simulink model "spike_generator_sim"  (R2020b)
settings: Solver=FixedStepDiscrete  StartTime=0.0  StopTime=stopTime  RelTol=1e-3
values from neighbouring files (symbols this model uses):
  nSites = 4    [modelparameters.m]
  tabs = 10e-3    (= 0.01)    [modelparameters.m]
  trel = 10e-3    (= 0.01)    [modelparameters.m]
undefined symbols (not defined in the file or in its folder): mp
libraries: dspsrcs4 x1
settings Model: Creator=Ross  LastModifiedBy=tyler
settings SolverCC: AutoInsertRateTranBlk=on
settings DataIOCC: ReturnWorkspaceOutputs=off
settings OptimizationCC: BlockReduction=off  ConditionallyExecuteInputs=off  DefaultParameterBehavior=Inlined
settings DebuggingCC: ReadBeforeWriteMsg=DisableAll  WriteAfterWriteMsg=DisableAll  WriteAfterReadMsg=DisableAll  AlgebraicLoopMsg=error  MultiTaskDSMMsg=none  SingleTaskRateTransMsg=error  PregeneratedLibrarySubsystemCodeDiagnostic=none  ArithmeticOperatorsInVariantConditions=warning
settings HardwareCC: ProdBitPerPointer=32  ProdBitPerSizeT=32  ProdBitPerPtrDiffT=32  ProdLargestAtomicFloat=None  ProdIntDivRoundTo=Undefined  ProdEndianess=Unspecified  ProdWordSize=32  ProdHWDeviceType=ASIC/FPGA->ASIC/FPGA  TargetBitPerPointer=64  TargetBitPerSizeT=64  TargetBitPerPtrDiffT=64  TargetLongLongMode=on  TargetIntDivRoundTo=Zero  TargetEndianess=LittleEndian  TargetWordSize=64  TargetHWDeviceType=Custom Processor->MATLAB Host Computer  ProdEqTarget=off
settings ModelReferenceCC: UpdateModelReferenceTargets=IfOutOfDate
settings SFSimCC: SFSimEcho=off  SimUseLocalCustomCode=off  CustomCodeUndefinedFunction=UseInterfaceOnly
settings RTWCC: RTWUseLocalCustomCode=off

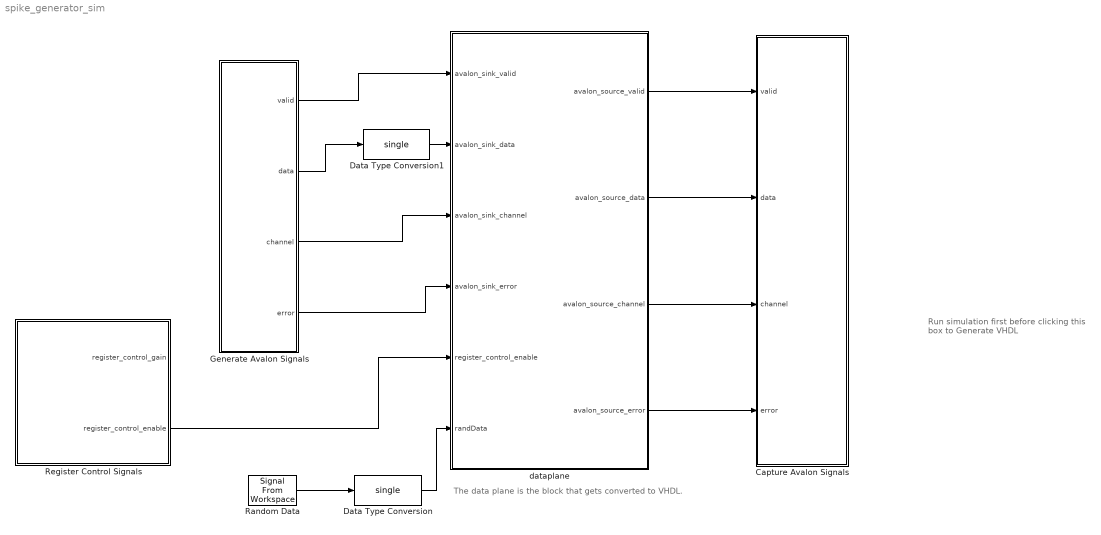
== system spike_generator_sim ==
  note: The data plane is the block that gets converted to VHDL.
  note: Run simulation first
      | before clicking this box to
      | Generate VHDL
  Capture Avalon Signals : Subsystem
  Data Type Conversion : DataTypeConversion  OutDataTypeStr=single
  Data Type Conversion1 : DataTypeConversion  OutDataTypeStr=single
  Generate Avalon Signals : Subsystem
  Random Data : dspsrcs4/Signal From Workspace  X=randNums  Ts=mp.Ts_sim  nsamps=1  OutputAfterFinalValue=Setting to zero  ignoreOrWarnInputAndFrameLengths=off  OutputFrames=off
  Register Control Signals : Subsystem
  dataplane : Subsystem  TreatAsAtomicUnit=on
  wires:
  Generate Avalon Signals/2(data) -> Data Type Conversion1/1
  Generate Avalon Signals/1(valid) -> dataplane/1(avalon_sink_valid)
  Generate Avalon Signals/3(channel) -> dataplane/3(avalon_sink_channel)
  Generate Avalon Signals/4(error) -> dataplane/4(avalon_sink_error)
  dataplane/2(avalon_source_data) -> Capture Avalon Signals/2(data)
  dataplane/1(avalon_source_valid) -> Capture Avalon Signals/1(valid)
  dataplane/3(avalon_source_channel) -> Capture Avalon Signals/3(channel)
  dataplane/4(avalon_source_error) -> Capture Avalon Signals/4(error)
  Register Control Signals/2(register_control_enable) -> dataplane/5(register_control_enable)
  Random Data/1 -> Data Type Conversion/1
  Data Type Conversion/1 -> dataplane/6(randData)
  Data Type Conversion1/1 -> dataplane/2(avalon_sink_data)

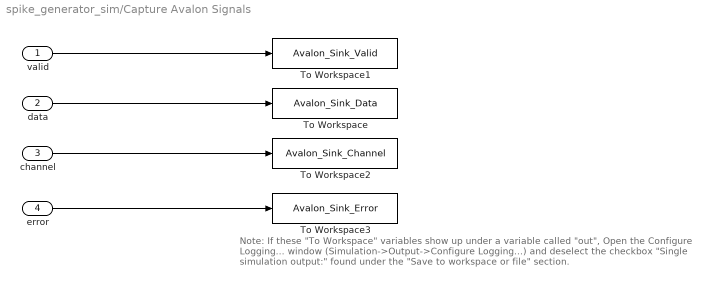
== system spike_generator_sim/Capture Avalon Signals ==
  note: Note:  If these "To Workspace" variables show up under a variable called "out",
      | Open the Configure Logging... window (Simulation->Output->Configure Logging...)
      | and deselect the checkbox "Single simulation output:" found under the "Save to workspace or file" section.
  valid : Inport
  data : Inport  Port=2
  channel : Inport  Port=3
  error : Inport  Port=4
  To Workspace : ToWorkspace  VariableName=Avalon_Sink_Data  SaveFormat=Timeseries  SampleTime=-1
  To Workspace1 : ToWorkspace  VariableName=Avalon_Sink_Valid  SaveFormat=Timeseries  SampleTime=-1
  To Workspace2 : ToWorkspace  VariableName=Avalon_Sink_Channel  SaveFormat=Timeseries  SampleTime=-1
  To Workspace3 : ToWorkspace  VariableName=Avalon_Sink_Error  SaveFormat=Timeseries  SampleTime=-1
  wires:
  data/1 -> To Workspace/1
  valid/1 -> To Workspace1/1
  error/1 -> To Workspace3/1
  channel/1 -> To Workspace2/1

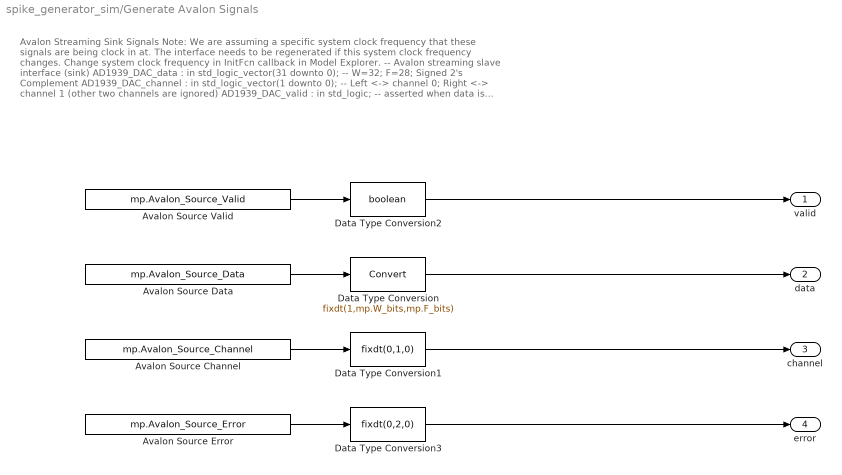
== system spike_generator_sim/Generate Avalon Signals ==
  note: Avalon Streaming Sink Signals
      | Note: We are assuming a specific system clock frequency that these signals are being clock in at.
      | The interface needs to be regenerated if this system clock frequency changes. Change system clock frequency in InitFcn callback in Model Explorer.
      |
      | -- Avalon streaming slave interface (sink)
      | AD1939_DAC_data : in std_logic_vector(31 downto 0); -- W=32; F=28; Signed 2's Complement
      | AD1939_DAC_channel : in std_logic_vector(1 downto 0); -- Left <-> channel 0; Right <-> channel 1 (other two channels are ignored)
      | AD1939_DAC_valid : in std_logic; -- asserted when data is valid
      | AD1939_DAC_error : in std_logic_vector(1 downto 0) -- error channel is ignored, assumed to be error free at this point
      |
      | For more information on the data-channel-valid protocol, s ee chapter 5 in Intel's Avalon Interfaced Specification (p. 40) at https://www.intel.com/content/dam/www/programmable/us/en/pdfs/literature/manual/mnl_avalon_spec.pdf
  Avalon Source Channel : FromWorkspace  VariableName=mp.Avalon_Source_Channel  OutDataTypeStr=double  SampleTime=mp.Ts_sim
  "Avalon Source Data " : FromWorkspace  VariableName=mp.Avalon_Source_Data  OutDataTypeStr=double  SampleTime=mp.Ts_sim
  Avalon Source Error : FromWorkspace  VariableName=mp.Avalon_Source_Error  OutDataTypeStr=double  SampleTime=mp.Ts_sim
  Avalon Source Valid : FromWorkspace  VariableName=mp.Avalon_Source_Valid  OutDataTypeStr=double  SampleTime=mp.Ts_sim
  Data Type Conversion : DataTypeConversion  OutDataTypeStr=fixdt(1,mp.W_bits,mp.F_bits)
  Data Type Conversion1 : DataTypeConversion  OutDataTypeStr=fixdt(0,1,0)
  Data Type Conversion2 : DataTypeConversion  OutDataTypeStr=boolean
  Data Type Conversion3 : DataTypeConversion  OutDataTypeStr=fixdt(0,2,0)
  valid : Outport  VectorParamsAs1DForOutWhenUnconnected=off
  data : Outport  Port=2  VectorParamsAs1DForOutWhenUnconnected=off
  channel : Outport  Port=3  VectorParamsAs1DForOutWhenUnconnected=off
  error : Outport  Port=4  VectorParamsAs1DForOutWhenUnconnected=off
  wires:
  Data Type Conversion1/1 -> channel/1
  Data Type Conversion2/1 -> valid/1
  Avalon Source Error/1 -> Data Type Conversion3/1
  Data Type Conversion/1 -> data/1
  Avalon Source Valid/1 -> Data Type Conversion2/1
  Data Type Conversion3/1 -> error/1
  Avalon Source Channel/1 -> Data Type Conversion1/1
  "Avalon Source Data "/1 -> Data Type Conversion/1

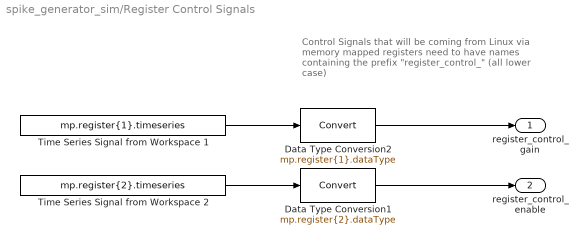
== system spike_generator_sim/Register Control Signals ==
  note: Control Signals that will be coming from Linux via
      | memory mapped registers need to have names
      | containing the prefix "register_control_"
      | (all lower case)
  Data Type Conversion1 : DataTypeConversion  OutDataTypeStr=mp.register{2}.dataType
  Data Type Conversion2 : DataTypeConversion  OutDataTypeStr=mp.register{1}.dataType
  Time Series Signal from Workspace 1 : FromWorkspace  VariableName=mp.register{1}.timeseries  OutDataTypeStr=double  SampleTime=mp.Ts_sim
  Time Series Signal from Workspace 2 : FromWorkspace  VariableName=mp.register{2}.timeseries  OutDataTypeStr=double  SampleTime=mp.Ts_sim
  register_control_gain : Outport  VectorParamsAs1DForOutWhenUnconnected=off
  register_control_enable : Outport  Port=2  VectorParamsAs1DForOutWhenUnconnected=off
  wires:
  Time Series Signal from Workspace 1/1 -> Data Type Conversion2/1
  Data Type Conversion2/1 -> register_control_gain/1
  Data Type Conversion1/1 -> register_control_enable/1
  Time Series Signal from Workspace 2/1 -> Data Type Conversion1/1

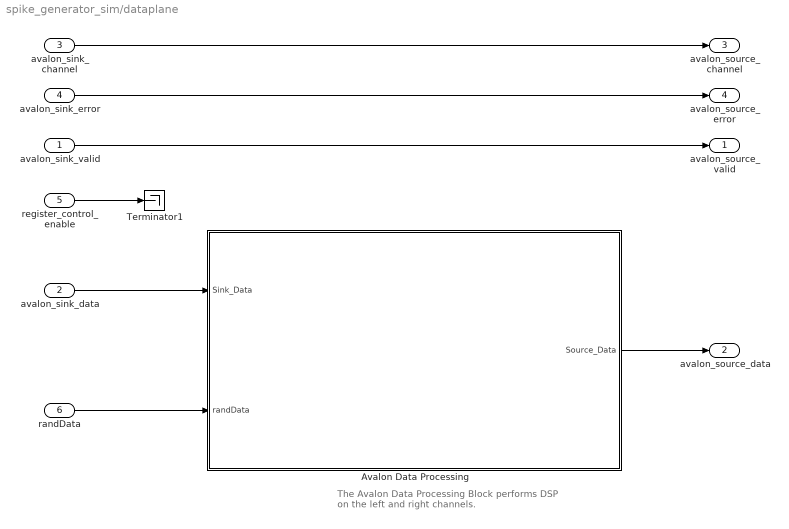
== system spike_generator_sim/dataplane ==
  note: The Avalon Data Processing Block
      | performs DSP on the left and right channels.
  avalon_sink_valid : Inport
  avalon_sink_data : Inport  Port=2
  avalon_sink_channel : Inport  Port=3
  avalon_sink_error : Inport  Port=4
  register_control_enable : Inport  Port=5
  randData : Inport  Port=6
  Avalon Data Processing : Subsystem  TreatAsAtomicUnit=on
  Terminator1 : Terminator
  avalon_source_valid : Outport  VectorParamsAs1DForOutWhenUnconnected=off
  avalon_source_data : Outport  Port=2  VectorParamsAs1DForOutWhenUnconnected=off
  avalon_source_channel : Outport  Port=3  VectorParamsAs1DForOutWhenUnconnected=off
  avalon_source_error : Outport  Port=4  VectorParamsAs1DForOutWhenUnconnected=off
  wires:
  avalon_sink_error/1 -> avalon_source_error/1
  Avalon Data Processing/1(Source_Data) -> avalon_source_data/1
  register_control_enable/1 -> Terminator1/1
  avalon_sink_valid/1 -> avalon_source_valid/1
  avalon_sink_channel/1 -> avalon_source_channel/1
  avalon_sink_data/1 -> Avalon Data Processing/1(Sink_Data)
  randData/1 -> Avalon Data Processing/2(randData)

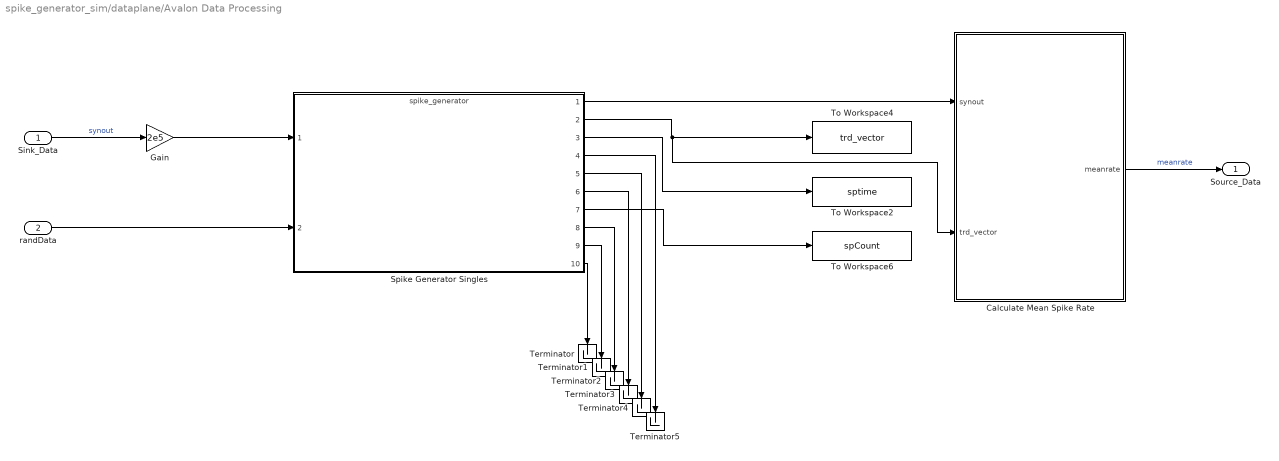
== system spike_generator_sim/dataplane/Avalon Data Processing ==
  Sink_Data : Inport
  randData : Inport  Port=2
  Calculate Mean Spike Rate : Subsystem
  Gain : Gain  Gain=2e5
  Spike Generator Singles : ModelReference  ModelNameDialog=spike_generator  SimulationMode=Normal  ModelReferenceVersion=1.255
  Terminator{,1..5} (6 alike) : Terminator
  To Workspace2 : ToWorkspace  VariableName=sptime  SampleTime=-1
      settings: Save2DSignal=2-D array (concatenate along first dimension)
  To Workspace4 : ToWorkspace  VariableName=trd_vector  SampleTime=-1
      settings: Save2DSignal=2-D array (concatenate along first dimension)
  To Workspace6 : ToWorkspace  VariableName=spCount  SampleTime=-1
      settings: Save2DSignal=2-D array (concatenate along first dimension)
  Source_Data : Outport  InitialOutput=0  VectorParamsAs1DForOutWhenUnconnected=off
  wires:
  Sink_Data/1 -> Gain/1  "synout"
  Spike Generator Singles/1 -> Calculate Mean Spike Rate/1(synout)
  randData/1 -> Spike Generator Singles/2
  Gain/1 -> Spike Generator Singles/1
  Spike Generator Singles/7 -> To Workspace6/1
  Calculate Mean Spike Rate/1(meanrate) -> Source_Data/1  "meanrate"
  Spike Generator Singles/2 -> Calculate Mean Spike Rate/2(trd_vector), To Workspace4/1
  Spike Generator Singles/3 -> To Workspace2/1
  Spike Generator Singles/10 -> Terminator/1
  Spike Generator Singles/9 -> Terminator1/1
  Spike Generator Singles/8 -> Terminator2/1
  Spike Generator Singles/6 -> Terminator3/1
  Spike Generator Singles/5 -> Terminator4/1
  Spike Generator Singles/4 -> Terminator5/1

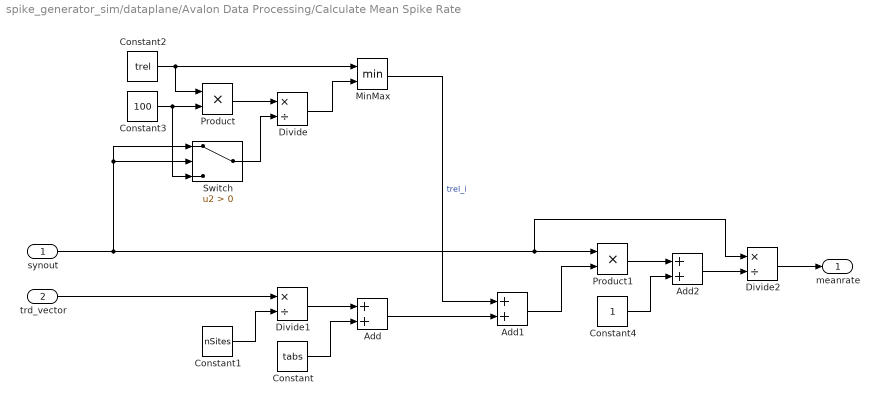
== system spike_generator_sim/dataplane/Avalon Data Processing/Calculate Mean Spike Rate ==
  synout : Inport
  trd_vector : Inport  Port=2
  Add : Sum
  Add1 : Sum
  Add2 : Sum
  Constant : Constant  Value=tabs  OutDataTypeStr=single  SampleTime=-1
  Constant1 : Constant  Value=nSites  OutDataTypeStr=single  SampleTime=-1
  Constant2 : Constant  Value=trel  OutDataTypeStr=single  SampleTime=-1
  Constant3 : Constant  Value=100  OutDataTypeStr=single  SampleTime=-1
  Constant4 : Constant  OutDataTypeStr=single  SampleTime=-1
  Divide : Product  Inputs=*/  RndMeth=Zero  SaturateOnIntegerOverflow=on
  Divide1 : Product  Inputs=*/  RndMeth=Zero  SaturateOnIntegerOverflow=on
  Divide2 : Product  Inputs=*/  RndMeth=Zero  SaturateOnIntegerOverflow=on
  MinMax : MinMax  Inputs=2
  Product : Product
  Product1 : Product
  Switch : Switch  Criteria=u2 > Threshold
  meanrate : Outport  VectorParamsAs1DForOutWhenUnconnected=off
  wires:
  Switch/1 -> Divide/2
  Divide2/1 -> meanrate/1
  Add2/1 -> Divide2/2
  Product1/1 -> Add2/1
  Add1/1 -> Product1/2
  Constant4/1 -> Add2/2
  Add/1 -> Add1/2
  Constant/1 -> Add/2
  Divide1/1 -> Add/1
  Constant1/1 -> Divide1/2
  MinMax/1 -> Add1/1  "trel_i"
  Divide/1 -> MinMax/2
  Product/1 -> Divide/1
  Constant3/1 -> Product/2, Switch/3
  Constant2/1 -> Product/1, MinMax/1
  trd_vector/1 -> Divide1/1
  synout/1 -> Product1/1, Divide2/1, Switch/2, Switch/1
